simulink model "Transmitter_16bit"  (R2017a)
settings: Solver=FixedStepDiscrete  StartTime=0.0  StopTime=10  RelTol=1e-3
InitFcn:
  | numHeaderBits = 16;
  | %numPreambleBits = 250;
  | AGCBarkerSymbols = 160+28;
  | EQTrainingSymbols = 250;
  | CRCGeneratorLag = 34; % CRCLen + 2
  | 
  | %% AGC Preamble
  | B13bipolar = [0 0 0 0 0 2 2 0 0 2 0 2];
  | rep = [B13bipolar, B13bipolar(1:4)];
  | AGCBarker = repmat(rep,1,10);
  | % Second preamble part
  | B11bipolar = [0 0 0 2 2 2 0 2  2 0 2];
  | TimingBarker = [B11bipolar,B11bipolar,B11bipolar,B11bipolar(1:6)];
  | PreambleBarkersInts = [AGCBarker, TimingBarker];
  | % Convert integer into their bit representation
  | PreambleBarkersBits = zeros(1,length(PreambleBarkersInts)*2);
  | PreambleBarkersBits(1:2:end) = (PreambleBarkersInts==2);
  | 
  | % Constants
  | % First preamble part
  | B13bipolar = [0 0 0 0 0 2 2 0 0 2 0 2];
  | rep = [B13bipolar, B13bipolar(1:4)];
  | AGCBarker = repmat(rep,1,10);
  | % Second preamble part
  | B11bipolar = [0 0 0 2 2 2 0 2  2 0 2];
  | TimingBarker = [B11bipolar,B11bipolar,B11bipolar(1:6)];
  | PreambleBarkersInts = [AGCBarker, TimingBarker];
  | % Convert integer into their bit representation
  | PreambleBarkersBits = false(1,length(PreambleBarkersInts)*2);
  | PreambleBarkersBits(1:2:end) = logical(PreambleBarkersInts==2);
  | pLen = uint16(length(PreambleBarkersBits));
libraries: simulink x11, hdlsllib x5, dspsigops x4, commseqgen3 x3, commdigbbndpm3 x2, commcnvcod2 x1, commcrc2 x1, commfilt2 x1
settings Model: DataTypeOverride=Off  Creator=tcollins  LastModifiedBy=tcollins
settings DataIOCC: SaveOutput=off  SaveTime=off
settings OptimizationCC: BlockReduction=off  ConditionallyExecuteInputs=off  DefaultParameterBehavior=Inlined
settings DebuggingCC: AlgebraicLoopMsg=error  SingleTaskRateTransMsg=error
settings HardwareCC: ProdBitPerPointer=32  ProdBitPerSizeT=32  ProdBitPerPtrDiffT=32  ProdLargestAtomicFloat=None  ProdIntDivRoundTo=Undefined  ProdEndianess=Unspecified  ProdWordSize=32  ProdHWDeviceType=ASIC/FPGA->ASIC/FPGA  ProdEqTarget=off

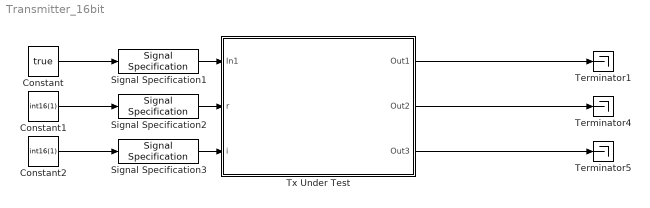
== system Transmitter_16bit ==
  Constant : Constant  Value=true  SampleTime=-1
  Constant1 : Constant  Value=int16(1)  SampleTime=-1
  Constant2 : Constant  Value=int16(1)  SampleTime=-1
  Signal Specification1 : SignalSpecification  OutDataTypeStr=boolean  SampleTime=1e-6
  Signal Specification2 : SignalSpecification  OutDataTypeStr=int16  SampleTime=1e-6
  Signal Specification3 : SignalSpecification  OutDataTypeStr=int16  SampleTime=1e-6
  Terminator1 : Terminator
  Terminator4 : Terminator
  Terminator5 : Terminator
  Tx Under Test : Subsystem  TreatAsAtomicUnit=on
  wires:
  Constant/1 -> Signal Specification1/1
  Tx Under Test/1(Out1) -> Terminator1/1
  Tx Under Test/2(Out2) -> Terminator4/1
  Tx Under Test/3(Out3) -> Terminator5/1
  Signal Specification1/1 -> Tx Under Test/1(In1)
  Constant1/1 -> Signal Specification2/1
  Signal Specification2/1 -> Tx Under Test/2("r ")
  Constant2/1 -> Signal Specification3/1
  Signal Specification3/1 -> Tx Under Test/3(i)

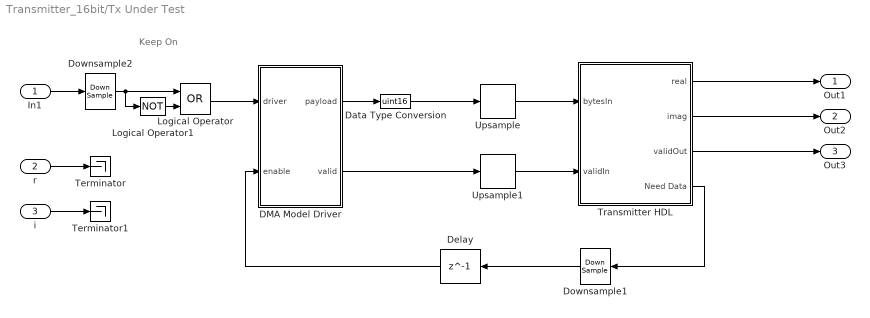
== system Transmitter_16bit/Tx Under Test ==
  note: Keep On
  In1 : Inport
  "r " : Inport  Port=2
  i : Inport  Port=3
  DMA Model Driver : MATLAB Function  TreatAsAtomicUnit=on
  Data Type Conversion : DataTypeConversion  OutDataTypeStr=uint16
  Delay : Delay  DelayLength=1
  Downsample1 : DownSample  N=4  RateOptions=Allow multirate processing
  Downsample2 : DownSample  N=4  RateOptions=Allow multirate processing
  Logical Operator : Logic  Operator=OR  AllPortsSameDT=off  OutDataTypeStr=boolean
  Logical Operator1 : Logic  Operator=NOT  AllPortsSameDT=off  OutDataTypeStr=boolean
  Terminator : Terminator
  Terminator1 : Terminator
  Transmitter HDL : Subsystem  TreatAsAtomicUnit=on
  Upsample : dspsigops/Upsample  N=4  phase=0  RateOptions=Allow multirate processing  ic=0  mode=Unused parameter value
  Upsample1 : dspsigops/Upsample  N=4  phase=0  RateOptions=Allow multirate processing  ic=0  mode=Unused parameter value
  Out1 : Outport
  Out2 : Outport  Port=2
  Out3 : Outport  Port=3
  wires:
  Transmitter HDL/4(Need Data) -> Downsample1/1
  Transmitter HDL/2(imag) -> Out2/1
  Transmitter HDL/1(real) -> Out1/1
  Transmitter HDL/3(validOut) -> Out3/1
  DMA Model Driver/1(payload) -> Data Type Conversion/1
  Delay/1 -> DMA Model Driver/2(enable)
  In1/1 -> Downsample2/1
  Data Type Conversion/1 -> Upsample/1
  DMA Model Driver/2(valid) -> Upsample1/1
  "r "/1 -> Terminator/1
  i/1 -> Terminator1/1
  Upsample/1 -> Transmitter HDL/1(bytesIn)
  Upsample1/1 -> Transmitter HDL/2(validIn)
  Downsample1/1 -> Delay/1
  Logical Operator/1 -> DMA Model Driver/1(driver)
  Logical Operator1/1 -> Logical Operator/2
  Downsample2/1 -> Logical Operator/1, Logical Operator1/1

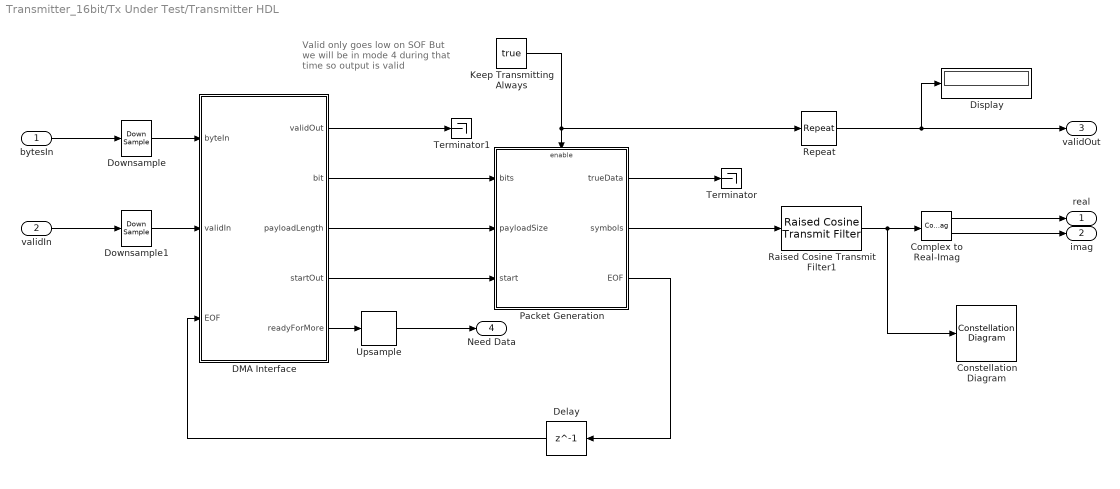
== system Transmitter_16bit/Tx Under Test/Transmitter HDL ==
  note: Valid only goes low on SOF
      | But we will be in mode 4 during
      | that time so output is valid
  bytesIn : Inport
  validIn : Inport  Port=2
  Complex to Real-Imag : ComplexToRealImag
  Constellation Diagram : ConstellationDiagram
  DMA Interface : Subsystem
  Delay : Delay  DelayLength=1
  Display : Display
  Downsample : DownSample  N=4  RateOptions=Allow multirate processing
  Downsample1 : DownSample  N=4  RateOptions=Allow multirate processing
  Keep Transmitting Always : Constant  Value=true  SampleTime=-1
  Packet Generation : Subsystem
  Raised Cosine Transmit Filter1 : commfilt2/Raised Cosine Transmit Filter  filtType=Square root  R=0.5  filtSpan=8  N=4  filterGain=1  RateOptions=Allow multirate processing  framing=Mute  checkCoeff=off  variableName=rcTxFilt1  checkGain=Normalized  sampMode=Mute  saveAsFlag=0  currentFiltSpan=8  D=(8)/2  launchFVT=on  roundingMode=Floor  overflowMode=off  coeffDataTypeStr=Inherit: Same word length as input  coeffMin=[]  coeffMax=[]  coeffLastDataTypeStr=Inherit: Same word length as input  outputMode=Binary point scaling  outputWordLength=16  outputFracLength=14  outputDataTypeStr=fixdt(1,16,14)  outputMin=[]  outputMax=[]  outputLastDataTypeStr=fixdt(1,16,14)
  Repeat : dspsigops/Repeat  N=4  InputProcessing=Columns as channels (frame based)  RateOptions=Allow multirate processing  ic=0  mode=Unused parameter value
      settings: SourceProductName=DSP System Toolbox
  Terminator : Terminator
  Terminator1 : Terminator
  Upsample : dspsigops/Upsample  N=4  phase=0  RateOptions=Allow multirate processing  ic=0  mode=Unused parameter value
  real : Outport
  imag : Outport  Port=2
  validOut : Outport  Port=3
  Need Data : Outport  Port=4
  wires:
  Raised Cosine Transmit Filter1/1 -> Constellation Diagram/1, Complex to Real-Imag/1
  Complex to Real-Imag/1 -> real/1
  Complex to Real-Imag/2 -> imag/1
  DMA Interface/2(bit) -> Packet Generation/1(bits)
  DMA Interface/3(payloadLength) -> Packet Generation/2(payloadSize)
  DMA Interface/4(startOut) -> Packet Generation/3(start)
  Packet Generation/2(symbols) -> Raised Cosine Transmit Filter1/1
  DMA Interface/5(readyForMore) -> Upsample/1
  Repeat/1 -> validOut/1, Display/1
  Packet Generation/1(trueData) -> Terminator/1
  Packet Generation/3(EOF) -> Delay/1
  Delay/1 -> DMA Interface/3(EOF)
  bytesIn/1 -> Downsample/1
  validIn/1 -> Downsample1/1
  Upsample/1 -> Need Data/1
  Downsample/1 -> DMA Interface/1(byteIn)
  Downsample1/1 -> DMA Interface/2(validIn)
  DMA Interface/1(validOut) -> Terminator1/1
  Keep Transmitting Always/1 -> Packet Generation/Enable, Repeat/1

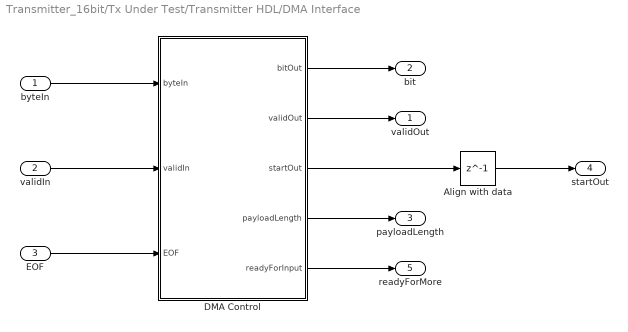
== system Transmitter_16bit/Tx Under Test/Transmitter HDL/DMA Interface ==
  byteIn : Inport
  validIn : Inport  Port=2
  EOF : Inport  Port=3
  Align with data : Delay  DelayLength=1
  DMA Control : MATLAB Function  TreatAsAtomicUnit=on
  validOut : Outport
  bit : Outport  Port=2
  payloadLength : Outport  Port=3  OutDataTypeStr=uint16
  startOut : Outport  Port=4
  readyForMore : Outport  Port=5
  wires:
  byteIn/1 -> DMA Control/1(byteIn)
  DMA Control/1(bitOut) -> bit/1
  DMA Control/5(readyForInput) -> readyForMore/1
  DMA Control/4(payloadLength) -> payloadLength/1
  DMA Control/2(validOut) -> validOut/1
  validIn/1 -> DMA Control/2(validIn)
  Align with data/1 -> startOut/1
  DMA Control/3(startOut) -> Align with data/1
  EOF/1 -> DMA Control/3(EOF)

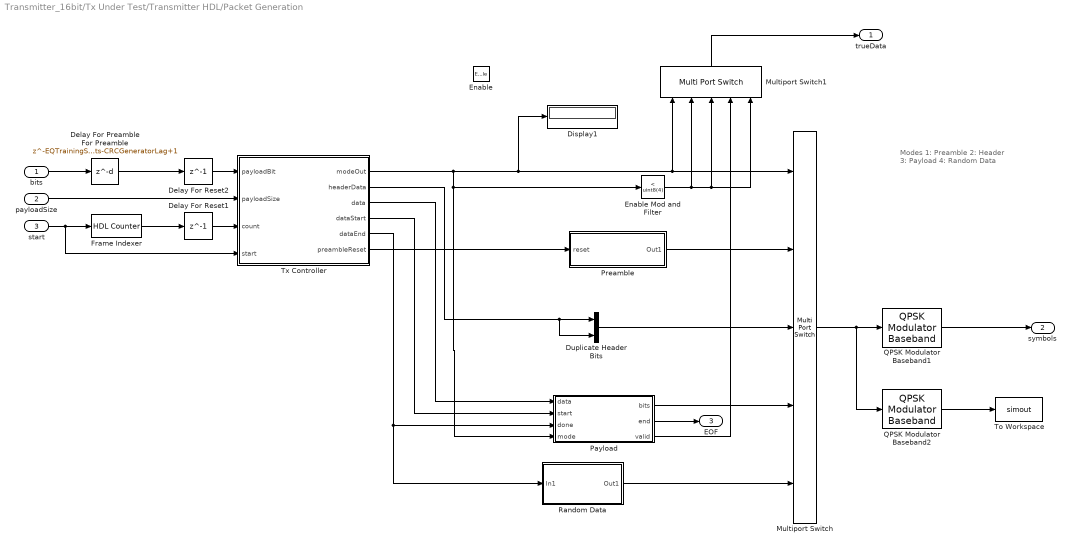
== system Transmitter_16bit/Tx Under Test/Transmitter HDL/Packet Generation ==
  note: Modes
      | 	1: Preamble
      | 	2: Header
      | 	3: Payload
      | 	4: Random Data
  bits : Inport  OutDataTypeStr=boolean
  payloadSize : Inport  Port=2
  start : Inport  Port=3
  Enable : EnablePort
  Delay For Preamble For Preamble : Delay  DelayLength=EQTrainingSymbols+AGCBarkerSymbols+numHeaderBits-CRCGeneratorLag+1  InitialCondition=false
  Delay For Reset1 : Delay  DelayLength=1
  Delay For Reset2 : Delay  DelayLength=1  InitialCondition=false
  Display1 : Display
  Duplicate Header Bits : Concatenate
  Enable Mod and Filter : simulink/Logic and Bit Operations/Compare To Constant  relop=<  const=uint8(4)  OutDataTypeStr=boolean
  Frame Indexer : hdlsllib/HDL Operations/HDL Counter  CountType=Count limited  CountInit=0  CountStep=1  CountMax=2^16+EQTrainingSymbols+AGCBarkerSymbols+numHeaderBits  CountFromType=Specify  CountFrom=0  CountResetPort=on  CountLoadPort=off  CountEnbPort=off  CountDirPort=off  CountDataType=Unsigned  CountWordLen=32  CountFracLen=0  CountSampTime=1
      settings: SourceProductName=HDL Coder  SourceProductBaseCode=HD
  Multiport Switch : MultiPortSwitch  Inputs=4
  Multiport Switch1 : MultiPortSwitch  Inputs=4
  Payload : Subsystem
  Preamble : Subsystem
  QPSK Modulator Baseband1 : commdigbbndpm3/QPSK Modulator Baseband  InType=Bit  Enc=Binary  Ph=pi/4  outDtype=Fixed-point  outWordLen=16  outUDDataType=sfix(16)  outFracLenMode=User-defined  outFracLen=15  outDataTypeStr=fixdt(1,16,15)  outLastDataTypeStr=fixdt(1,16,15)
  QPSK Modulator Baseband2 : commdigbbndpm3/QPSK Modulator Baseband  InType=Bit  Enc=Binary  Ph=pi/4  outDtype=double  outWordLen=16  outUDDataType=sfix(16)  outFracLenMode=User-defined  outFracLen=15  outDataTypeStr=double  outLastDataTypeStr=double
  Random Data : Subsystem
  To Workspace : ToWorkspace  VariableName=simout  SaveFormat=Timeseries  SampleTime=-1
  Tx Controller : MATLAB Function  TreatAsAtomicUnit=on
  trueData : Outport  InitialOutput=0
  symbols : Outport  Port=2  InitialOutput=complex(0)
  EOF : Outport  Port=3  OutDataTypeStr=boolean  InitialOutput=0
  wires:
  Tx Controller/2(headerData) -> Duplicate Header Bits/2, Duplicate Header Bits/1
  Random Data/1(Out1) -> Multiport Switch/5
  Enable Mod and Filter/1 -> Multiport Switch1/5, Multiport Switch1/3, Multiport Switch1/2
  Tx Controller/3(data) -> Payload/1(data)
  Tx Controller/4(dataStart) -> Payload/2(start)
  Delay For Preamble For Preamble/1 -> Delay For Reset2/1
  start/1 -> Tx Controller/4(start), Frame Indexer/1
  Preamble/1(Out1) -> Multiport Switch/2
  bits/1 -> Delay For Preamble For Preamble/1
  QPSK Modulator Baseband1/1 -> symbols/1
  Multiport Switch1/1 -> trueData/1
  Delay For Reset1/1 -> Tx Controller/3(count)
  Multiport Switch/1 -> QPSK Modulator Baseband2/1, QPSK Modulator Baseband1/1
  Tx Controller/5(dataEnd) -> Payload/3(done), Random Data/1(In1)
  Payload/1(bits) -> Multiport Switch/4
  Duplicate Header Bits/1 -> Multiport Switch/3
  Frame Indexer/1 -> Delay For Reset1/1
  Payload/3(valid) -> Multiport Switch1/4
  Payload/2(end) -> EOF/1
  payloadSize/1 -> Tx Controller/2(payloadSize)
  Tx Controller/1(modeOut) -> Display1/1, Multiport Switch/1, Multiport Switch1/1, Payload/4(mode), Enable Mod and Filter/1
  Tx Controller/6(preambleReset) -> Preamble/1(reset)
  Delay For Reset2/1 -> Tx Controller/1(payloadBit)
  QPSK Modulator Baseband2/1 -> To Workspace/1

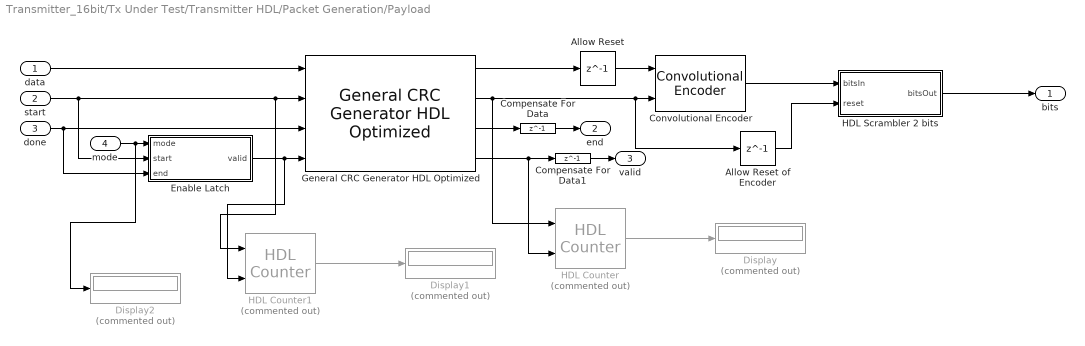
== system Transmitter_16bit/Tx Under Test/Transmitter HDL/Packet Generation/Payload ==
  data : Inport
  start : Inport  Port=2
  done : Inport  Port=3
  mode : Inport  Port=4
  Allow Reset : Delay  DelayLength=1
  Allow Reset of Encoder : Delay  DelayLength=1
  Compensate For Data : Delay  DelayLength=1
  Compensate For Data1 : Delay  DelayLength=1
  Convolutional Encoder : commcnvcod2/Convolutional Encoder  trellis=poly2trellis(7, [171 133])  opMode=Reset on nonzero input via port  DelayedResetAction=on  hasIniStPort=off  hasFinStPort=off  usePuncVector=off  punctureVector=[1; 1; 0; 1; 0; 1]  reset=Unused parameter value
      settings: SourceProductName=Communications System Toolbox  SourceProductBaseCode=CM
  Display : Display  Commented=on
  Display1 : Display  Commented=on
  Display2 : Display  Commented=on
  Enable Latch : Subsystem
  General CRC Generator HDL Optimized : commcrc2/General CRC Generator HDL Optimized  Polynomial=[1 0 0 0 0 0 1 0 0 1 1 0 0 0 0 0 1 0 0 0 1 1 1 0 1 1 0 1 1 0 1 1 1]  InitialState=0  DirectMethod=off  ReflectInput=off  ReflectCRCChecksum=off  FinalXORValue=0  SimulateUsing=Code generation
      settings: SourceProductName=Communications System Toolbox  SourceProductBaseCode=CM
  HDL Counter : hdlsllib/HDL Operations/HDL Counter  Commented=on  CountType=Count limited  CountInit=0  CountStep=1  CountMax=1e4  CountFromType=Initial value  CountFrom=0  CountResetPort=on  CountLoadPort=off  CountEnbPort=on  CountDirPort=off  CountDataType=Unsigned  CountWordLen=16  CountFracLen=0  CountSampTime=1
      settings: SourceProductName=HDL Coder  SourceProductBaseCode=HD
  HDL Counter1 : hdlsllib/HDL Operations/HDL Counter  Commented=on  CountType=Count limited  CountInit=0  CountStep=1  CountMax=1e4  CountFromType=Initial value  CountFrom=0  CountResetPort=on  CountLoadPort=off  CountEnbPort=on  CountDirPort=off  CountDataType=Unsigned  CountWordLen=16  CountFracLen=0  CountSampTime=1
      settings: SourceProductName=HDL Coder  SourceProductBaseCode=HD
  HDL Scrambler 2 bits : Subsystem  mask{poly=[1 1 0 1 0 1 0 1], init_state=[0 1 0 0 0 1 0]}
      mask prompts: poly "Polynomial"; init_state "Initial State"
  bits : Outport
  end : Outport  Port=2
  valid : Outport  Port=3
  wires:
  General CRC Generator HDL Optimized/1 -> Allow Reset/1
  data/1 -> General CRC Generator HDL Optimized/1
  start/1 -> Enable Latch/2(start), HDL Counter1/1, General CRC Generator HDL Optimized/2
  General CRC Generator HDL Optimized/4 -> HDL Counter/2, Compensate For Data1/1
  done/1 -> Enable Latch/3(end), General CRC Generator HDL Optimized/3
  mode/1 -> Display2/1, Enable Latch/1(mode)
  Convolutional Encoder/1 -> HDL Scrambler 2 bits/1(bitsIn)
  General CRC Generator HDL Optimized/2 -> HDL Counter/1, Allow Reset of Encoder/1, Convolutional Encoder/2
  HDL Scrambler 2 bits/1(bitsOut) -> bits/1
  Enable Latch/1(valid) -> HDL Counter1/2, General CRC Generator HDL Optimized/4
  Allow Reset/1 -> Convolutional Encoder/1
  General CRC Generator HDL Optimized/3 -> Compensate For Data/1
  Allow Reset of Encoder/1 -> HDL Scrambler 2 bits/2(reset)
  HDL Counter/1 -> Display/1
  HDL Counter1/1 -> Display1/1
  Compensate For Data/1 -> end/1
  Compensate For Data1/1 -> valid/1

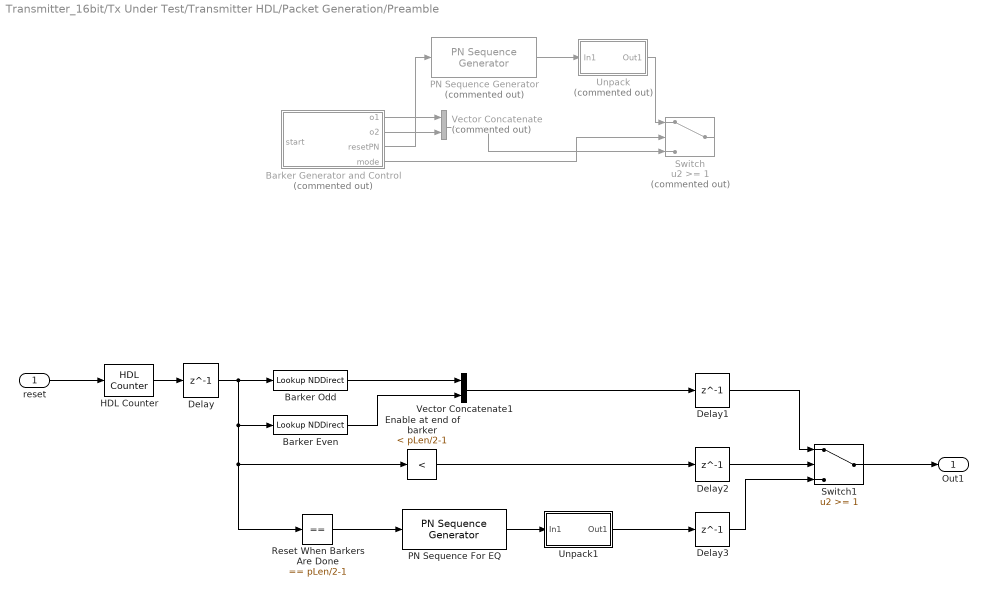
== system Transmitter_16bit/Tx Under Test/Transmitter HDL/Packet Generation/Preamble ==
  reset : Inport
  Barker Even : LookupNDDirect  NumberOfTableDimensions=1  Table=[PreambleBarkersBits(4:2:end),false(1,400)]  DiagnosticForOutOfRangeInput=Error  TableDataTypeStr=boolean
  Barker Generator and Control : MATLAB Function  Commented=on  TreatAsAtomicUnit=on
  Barker Odd : LookupNDDirect  NumberOfTableDimensions=1  Table=[PreambleBarkersBits(3:2:end-1),false(1,400)]  DiagnosticForOutOfRangeInput=Error  TableDataTypeStr=boolean
  Delay{,1..3} (4 alike) : Delay  DelayLength=1
  Enable at end of barker : simulink/Logic and Bit Operations/Compare To Constant  relop=<  const=pLen/2-1  OutDataTypeStr=boolean
  HDL Counter : hdlsllib/HDL Operations/HDL Counter  CountType=Count limited  CountInit=0  CountStep=1  CountMax=pLen/2-2+400  CountFromType=Initial value  CountFrom=0  CountResetPort=on  CountLoadPort=off  CountEnbPort=off  CountDirPort=off  CountDataType=Unsigned  CountWordLen=16  CountFracLen=0  CountSampTime=1
      settings: SourceProductName=HDL Coder  SourceProductBaseCode=HD
  PN Sequence For EQ : commseqgen3/PN Sequence Generator  poly='z^5 + z^3 + z^1 + 1'  ini_sta=[1 1 1 0 0]  outBitMaskSource=Dialog parameter  shift=0  outVarSiz=off  maxOutSizeMode=Dialog parameter  maxOutSize=[10 1]  Ts=-1  sampPerFrame=1  reset=on  bitPackedOutputs=on  outDataType=double  numPackedBits=2  bitPackDataSigned=off  bitPackedOutDType=Smallest integer
      settings: SourceProductName=Communications System Toolbox
  PN Sequence Generator : commseqgen3/PN Sequence Generator  Commented=on  poly='z^3 + z^2 + 1'  ini_sta=[0 0 1]  outBitMaskSource=Dialog parameter  shift=0  outVarSiz=off  maxOutSizeMode=Dialog parameter  maxOutSize=[10 1]  Ts=-1  sampPerFrame=1  reset=on  bitPackedOutputs=on  outDataType=double  numPackedBits=2  bitPackDataSigned=off  bitPackedOutDType=Smallest integer
      settings: SourceProductName=Communications System Toolbox
  Reset When Barkers Are Done : simulink/Logic and Bit Operations/Compare To Constant  relop===  const=pLen/2-1  OutDataTypeStr=boolean
  Switch : Switch  Commented=on  Threshold=1
  Switch1 : Switch  Threshold=1
  Unpack : Subsystem  Commented=on
  Unpack1 : Subsystem
  Vector Concatenate : Concatenate  Commented=on
  Vector Concatenate1 : Concatenate
  Out1 : Outport
  wires:
  reset/1 -> HDL Counter/1
  Barker Odd/1 -> Vector Concatenate1/1
  Barker Even/1 -> Vector Concatenate1/2
  PN Sequence For EQ/1 -> Unpack1/1(In1)
  Switch1/1 -> Out1/1
  Reset When Barkers Are Done/1 -> PN Sequence For EQ/1
  Barker Generator and Control/3(resetPN) -> PN Sequence Generator/1
  Barker Generator and Control/1(o1) -> Vector Concatenate/1
  Barker Generator and Control/4(mode) -> Switch/2
  PN Sequence Generator/1 -> Unpack/1(In1)
  Barker Generator and Control/2(o2) -> Vector Concatenate/2
  Unpack/1(Out1) -> Switch/1
  Vector Concatenate/1 -> Switch/3
  ? -> Barker Generator and Control/1(start)
  HDL Counter/1 -> Delay/1
  Delay/1 -> Enable at end of barker/1, Reset When Barkers Are Done/1, Barker Even/1, Barker Odd/1
  Vector Concatenate1/1 -> Delay1/1
  Enable at end of barker/1 -> Delay2/1
  Unpack1/1(Out1) -> Delay3/1
  Delay1/1 -> Switch1/1
  Delay2/1 -> Switch1/2
  Delay3/1 -> Switch1/3

== system Transmitter_16bit/Tx Under Test/Transmitter HDL/Packet Generation/Random Data ==
  In1 : Inport
  Random Data Gen : commseqgen3/PN Sequence Generator  poly='z^3 + z^2 + 1'  ini_sta=[0 0 1]  outBitMaskSource=Dialog parameter  shift=0  outVarSiz=off  maxOutSizeMode=Dialog parameter  maxOutSize=[10 1]  Ts=-1  sampPerFrame=1  reset=on  bitPackedOutputs=on  outDataType=double  numPackedBits=2  bitPackDataSigned=off  bitPackedOutDType=Smallest integer
      settings: SourceProductName=Communications System Toolbox
  Unpack : Subsystem
  Out1 : Outport
  wires:
  In1/1 -> Random Data Gen/1
  Unpack/1(Out1) -> Out1/1
  Random Data Gen/1 -> Unpack/1(In1)

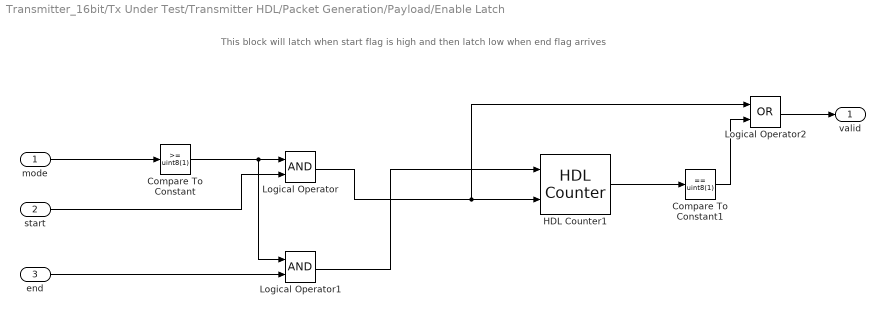
== system Transmitter_16bit/Tx Under Test/Transmitter HDL/Packet Generation/Payload/Enable Latch ==
  note: This block will latch when start flag is high and then latch low when end flag arrives
  mode : Inport
  start : Inport  Port=2
  end : Inport  Port=3
  Compare To Constant : simulink/Logic and Bit Operations/Compare To Constant  relop=>=  const=uint8(1)  OutDataTypeStr=boolean
  Compare To Constant1 : simulink/Logic and Bit Operations/Compare To Constant  relop===  const=uint8(1)  OutDataTypeStr=boolean
  HDL Counter1 : hdlsllib/HDL Operations/HDL Counter  CountType=Count limited  CountInit=0  CountStep=1  CountMax=1  CountFromType=Initial value  CountFrom=0  CountResetPort=on  CountLoadPort=off  CountEnbPort=on  CountDirPort=off  CountDataType=Unsigned  CountWordLen=8  CountFracLen=0  CountSampTime=1
      settings: SourceProductName=HDL Coder  SourceProductBaseCode=HD
  Logical Operator : Logic  AllPortsSameDT=off  OutDataTypeStr=boolean
  Logical Operator1 : Logic  AllPortsSameDT=off  OutDataTypeStr=boolean
  Logical Operator2 : Logic  Operator=OR  AllPortsSameDT=off  OutDataTypeStr=boolean
  valid : Outport
  wires:
  mode/1 -> Compare To Constant/1
  Compare To Constant/1 -> Logical Operator1/1, Logical Operator/1
  start/1 -> Logical Operator/2
  end/1 -> Logical Operator1/2
  HDL Counter1/1 -> Compare To Constant1/1
  Logical Operator1/1 -> HDL Counter1/1
  Logical Operator/1 -> Logical Operator2/1, HDL Counter1/2
  Compare To Constant1/1 -> Logical Operator2/2
  Logical Operator2/1 -> valid/1

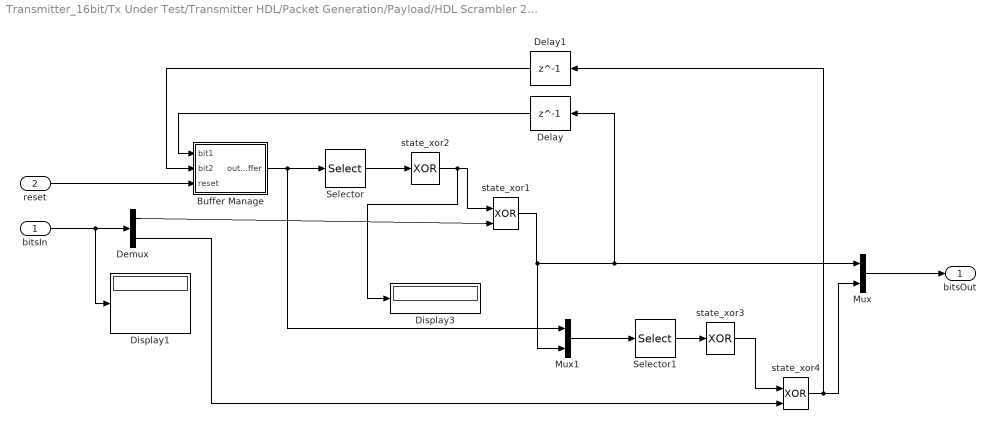
== system Transmitter_16bit/Tx Under Test/Transmitter HDL/Packet Generation/Payload/HDL Scrambler 2 bits ==
  bitsIn : Inport
  reset : Inport  Port=2
  Buffer Manage : MATLAB Function  TreatAsAtomicUnit=on
  Delay : Delay  DelayLength=1  InitialCondition=false
  Delay1 : Delay  DelayLength=1  InitialCondition=false
  Demux : Demux  Outputs=2
  Display1 : Display
  Display3 : Display
  Mux : Mux  Inputs=2
  Mux1 : Mux  Inputs=2
  Selector : Selector  IndexOptions=Index vector (dialog)  Indices=find(poly(2:end))  OutputSizes=1
  Selector1 : Selector  IndexOptions=Index vector (dialog)  Indices=1+find(poly(2:end))  OutputSizes=1
  state_xor1 : Logic  Operator=XOR  IconShape=distinctive  AllPortsSameDT=off  OutDataTypeStr=boolean
  state_xor2 : Logic  Operator=XOR  Inputs=1  IconShape=distinctive  AllPortsSameDT=off  OutDataTypeStr=boolean
  state_xor3 : Logic  Operator=XOR  Inputs=1  IconShape=distinctive  AllPortsSameDT=off  OutDataTypeStr=boolean
  state_xor4 : Logic  Operator=XOR  IconShape=distinctive  AllPortsSameDT=off  OutDataTypeStr=boolean
  bitsOut : Outport
  wires:
  bitsIn/1 -> Display1/1, Demux/1
  Selector/1 -> state_xor2/1
  state_xor2/1 -> Display3/1, state_xor1/1
  Demux/1 -> state_xor1/2
  state_xor1/1 -> Mux1/2, Mux/1, Delay/1
  Mux/1 -> bitsOut/1
  Mux1/1 -> Selector1/1
  Buffer Manage/1(outBuffer) -> Mux1/1, Selector/1
  Selector1/1 -> state_xor3/1
  state_xor3/1 -> state_xor4/1
  Demux/2 -> state_xor4/2
  state_xor4/1 -> Delay1/1, Mux/2
  Delay/1 -> Buffer Manage/1(bit1)
  reset/1 -> Buffer Manage/3(reset)
  Delay1/1 -> Buffer Manage/2(bit2)

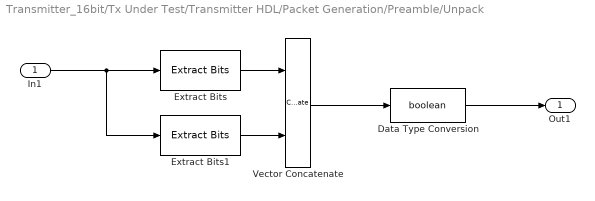
== system Transmitter_16bit/Tx Under Test/Transmitter HDL/Packet Generation/Preamble/Unpack ==
  In1 : Inport
  Data Type Conversion : DataTypeConversion  OutDataTypeStr=boolean
  Extract Bits : simulink/Logic and Bit Operations/Extract Bits  bitsToExtract=Range of bits  numBits=8  bitIdxRange=[1]  outScalingMode=Treat bit field as an integer
      settings: SourceProductName=Simulink
  Extract Bits1 : simulink/Logic and Bit Operations/Extract Bits  bitsToExtract=Range of bits  numBits=8  bitIdxRange=[0]  outScalingMode=Treat bit field as an integer
      settings: SourceProductName=Simulink
  Vector Concatenate : Concatenate
  Out1 : Outport
  wires:
  In1/1 -> Extract Bits1/1, Extract Bits/1
  Extract Bits/1 -> Vector Concatenate/1
  Extract Bits1/1 -> Vector Concatenate/2
  Vector Concatenate/1 -> Data Type Conversion/1
  Data Type Conversion/1 -> Out1/1

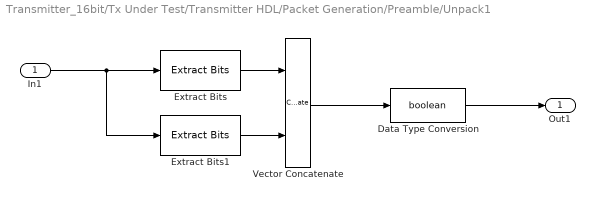
== system Transmitter_16bit/Tx Under Test/Transmitter HDL/Packet Generation/Preamble/Unpack1 ==
  In1 : Inport
  Data Type Conversion : DataTypeConversion  OutDataTypeStr=boolean
  Extract Bits : simulink/Logic and Bit Operations/Extract Bits  bitsToExtract=Range of bits  numBits=8  bitIdxRange=[1]  outScalingMode=Treat bit field as an integer
      settings: SourceProductName=Simulink
  Extract Bits1 : simulink/Logic and Bit Operations/Extract Bits  bitsToExtract=Range of bits  numBits=8  bitIdxRange=[0]  outScalingMode=Treat bit field as an integer
      settings: SourceProductName=Simulink
  Vector Concatenate : Concatenate
  Out1 : Outport
  wires:
  In1/1 -> Extract Bits1/1, Extract Bits/1
  Extract Bits/1 -> Vector Concatenate/1
  Extract Bits1/1 -> Vector Concatenate/2
  Vector Concatenate/1 -> Data Type Conversion/1
  Data Type Conversion/1 -> Out1/1

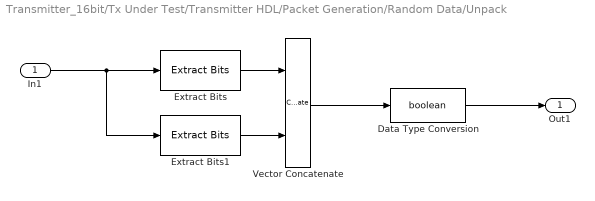
== system Transmitter_16bit/Tx Under Test/Transmitter HDL/Packet Generation/Random Data/Unpack ==
  In1 : Inport
  Data Type Conversion : DataTypeConversion  OutDataTypeStr=boolean
  Extract Bits : simulink/Logic and Bit Operations/Extract Bits  bitsToExtract=Range of bits  numBits=8  bitIdxRange=[0]  outScalingMode=Treat bit field as an integer
      settings: SourceProductName=Simulink
  Extract Bits1 : simulink/Logic and Bit Operations/Extract Bits  bitsToExtract=Range of bits  numBits=8  bitIdxRange=[1]  outScalingMode=Treat bit field as an integer
      settings: SourceProductName=Simulink
  Vector Concatenate : Concatenate
  Out1 : Outport
  wires:
  In1/1 -> Extract Bits1/1, Extract Bits/1
  Extract Bits/1 -> Vector Concatenate/1
  Extract Bits1/1 -> Vector Concatenate/2
  Vector Concatenate/1 -> Data Type Conversion/1
  Data Type Conversion/1 -> Out1/1

== matlab function Transmitter_16bit/Tx Under Test/Transmitter HDL/Packet Generation/Preamble/Barker Generator and Control ==
  data: start input; o1 output; o2 output; resetPN output; mode output
function [o1,o2,resetPN,mode] = fcn(start)

persistent indx

% Constants
% First preamble part
B13bipolar = [0 0 0 0 0 2 2 0 0 2 0 2];
rep = [B13bipolar, B13bipolar(1:4)];
AGCBarker = repmat(rep,1,10);
% Second preamble part
B11bipolar = [0 0 0 2 2 2 0 2  2 0 2];
TimingBarker = [B11bipolar,B11bipolar,B11bipolar(1:6)];
PreambleBarkersInts = [AGCBarker, TimingBarker];
% Convert integer into their bit representation
PreambleBarkersBits = false(1,length(PreambleBarkersInts)*2);
PreambleBarkersBits(1:2:end) = logical(PreambleBarkersInts==2);
pLen = uint16(length(PreambleBarkersBits));

% Async
if isempty(indx)
       indx = uint16(3);
end

% Reset and Async
if start
    resetPN = false; % Not important
    indx = uint16(3);
    o1 = PreambleBarkersBits(1);
    o2 = PreambleBarkersBits(2);
    mode = uint8(0); % Barker
else
    % Preamble is done, now PN can go
    if indx==(pLen+uint16(1))
        indx = indx + uint16(2); % Push last if to else
        resetPN = true;
    else
        resetPN = false;
    end
    % mode -> 0==Barkers | 1==PN
    if indx<(pLen)
        o1 = PreambleBarkersBits(indx);
        o2 = PreambleBarkersBits(indx+1);
        indx = indx + uint16(2);
        mode = uint8(0); % Barker
    else
        o1 = false;
        o2 = false;
        mode = uint8(1);
    end

%     if indx<pLen
%         o1 = PreambleBarkersBits(indx);
%         o2 = PreambleBarkersBits(indx+1);
%         indx = indx + uint16(2);
%         mode = uint8(0); % Barker
    
    
    
    
end

== matlab function Transmitter_16bit/Tx Under Test/Transmitter HDL/Packet Generation/Tx Controller ==
  data: modeOut output; headerData output; data output; payloadBit input; payloadSize input; count input; start input; dataStart output; dataEnd output; preambleReset output
function [modeOut, headerData, data, dataStart, dataEnd, preambleReset] = fcn(payloadBit,payloadSize,count, start)

% When we get a start flag buffers are reset and the next cycle with start
% in mode 0

% Reset: New payload size is passed at an int16
% 


persistent  headerBits numPayloadBits mode

numHeaderBits = uint32(16);
AGCBarkerSymbols = 160+28;
EQTrainingSymbols = 250; % 2 bits per symbol => 250 symbols
preambleBits = uint32(EQTrainingSymbols+AGCBarkerSymbols-0);
CRCLength = 32;
CRCGeneratorLag = CRCLength+2+0; % additional 1 is from reset of encoder
CodeRate = 2;
lagBits = 40+68;

% Async/Init
if isempty(numPayloadBits)
    % Sizes of frame sections
    numPayloadBits = uint32(0); 
    %headerBits = zeros(1,numHeaderBits)>0;
    headerBits = uint16(0);
    mode = uint8(4);
end

% Synchronous
switch mode
    case uint8(0) % Reset
        % Move to next mode on next input/clock
        mode = uint8(1);
        % Convert payloadSize to bits
        numPayloadBits = uint32(bitshift(payloadSize,3)+CRCLength);
        %headerBits = logical(bitget(CodeRate*(payloadSize+CRCLength),1:numHeaderBits));
        headerBits = uint16(bitshift((bitshift(payloadSize,3)+CRCLength+lagBits),1));        
        % Set outputs
        modeOut = uint8(4);
        headerData = false;
        data = false; % Not used downstream
        dataStart = false;
        dataEnd = false;
        preambleReset = true;
    case uint8(1) % Preamble
        % Set Next Mode
        if count>=(preambleBits)
            preambleReset = false;
            mode = uint8(2);
        elseif count==uint32(1)
            preambleReset = false;
            mode = uint8(1);
        else
            preambleReset = false;
            mode = uint8(1);
        end
        % Set outputs
        modeOut = uint8(1);
        headerData = false;
        % Start outputing data early to compensate for CRC lag
        if count>=(preambleBits+numHeaderBits-CRCGeneratorLag)
           data = payloadBit;
           % Set flag on first payload bit
           dataStart = count == (preambleBits+numHeaderBits-CRCGeneratorLag);
        else
           data = false;         
           dataStart = false;
        end
        dataEnd = false;
    case uint8(2) % Header bits
        % Set Next Mode
        if count>=(preambleBits+numHeaderBits)
            mode = uint8(3);
        else
            mode = uint8(2);
        end
        % Set outputs
        modeOut = uint8(2);
        %headerData = headerBits(count-preambleBits);
        headerData = bitget(headerBits,count-preambleBits)>0;
        data = payloadBit;
        dataStart = false;
        dataEnd = false;
        preambleReset = false;
    case uint8(3) % Payload bits and CRC
        % Set Next Mode
        if count>=(preambleBits+numHeaderBits+numPayloadBits)%+CRCGeneratorLag)
            % Will coencide with last CRC Bit
            mode = uint8(4);
        else
            mode = uint8(3);
        end
        % Set outputs
        modeOut = uint8(3);        
        headerData = false;
        data = payloadBit;
        % Set flag on last payload bit
        dataStart = false;
        dataEnd =   ( count==(preambleBits+numHeaderBits+numPayloadBits-CRCLength-CRCGeneratorLag-1) );
        preambleReset = false;
    otherwise %case uint8(4) % Waiting for data
        % Chilling for new start
        if start
           mode = uint8(0); 
        else
           mode = uint8(4);
        end
        % Set outputs
        modeOut = uint8(4);
        headerData = false;
        data = false; % Not used downstream
        dataStart = false;
        dataEnd = false;
        preambleReset = false;
end

== matlab function Transmitter_16bit/Tx Under Test/Transmitter HDL/DMA Interface/DMA Control ==
  data: byteIn input; bitOut output; validIn input; validOut output; startOut output; payloadLength output; readyForInput output; EOF input
function [bitOut,validOut,startOut,payloadLength,readyForInput] = DMA_Control(byteIn,validIn,EOF)

% This block converts the byte input pipeline into bits and extract the
% length the packet into its own signal

persistent wordBuffer bitCounter payloadLenBuff mode inputByteCounter

bitsInInput = uint8(16);
bytesInInput = uint16(2);

if isempty(wordBuffer)
    wordBuffer = uint16(0); % Must match number of bits defined by bitsInInput
    bitCounter = uint8(0);
    payloadLenBuff = uint16(0);
    mode = uint8(0);
    inputByteCounter = uint16(0);
end

%% Payload length setup
% Capture first payload length byte(s)
if validIn && mode == uint8(0)
    mode = uint8(2);
    payloadLenBuff = uint16(byteIn);
    % Set outputs
    bitOut = false;
    validOut = false;
    startOut = true;
    payloadLength = uint16(0);
    readyForInput = true;
    % Reset counters
    inputByteCounter = bytesInInput;% Reset
    bitCounter = uint8(1);% Reset
    
%% Payload output
elseif (bitCounter > uint8(0))  && (mode==uint8(2))
    % Set outputs
    if bitCounter==uint8(1)
        bitOut = bitget(byteIn,1)>0;
        wordBuffer = byteIn; % Save byte
    else
        bitOut = bitget(wordBuffer,bitCounter)>0;
    end
    startOut = false;
    payloadLength = uint16(payloadLenBuff);
    validOut = true;
    % Set flag to DMA and next mode
    if bitCounter >= uint8(bitsInInput)
        bitCounter = uint8(1); % Reset
        % If we've processed all the bytes we need to wait for downstream
        % to be done
        if inputByteCounter<payloadLenBuff
            readyForInput = true; % Tell them we need next byte
            % Bytes processed
            inputByteCounter = inputByteCounter + bytesInInput;    
        else
            readyForInput = false; % Hold DMA off for now, next call will go to EOF
            mode = uint8(3);
        end
    else
        bitCounter = bitCounter+uint8(1);
        readyForInput = false;
    end
% Waiting for EOF from packet generation
elseif (mode==uint8(3))
    bitOut = false;
    validOut = true; % Keep downstream processing going
    startOut = false;
    payloadLength = uint16(payloadLenBuff);
    if EOF % Done with frame now ask for more data
        readyForInput = true;
        mode = uint8(0);% Reset
    else
        readyForInput = false;
    end
    
else % not-valid and need another byte
    bitOut = false;
    if mode == uint8(0)
        validOut = true; % Let LFSR Run
    else
        validOut = false;
    end
    startOut = false;
    payloadLength = uint16(0);
    readyForInput = true;
end

== matlab function Transmitter_16bit/Tx Under Test/Transmitter HDL/Packet Generation/Payload/HDL Scrambler 2 bits/Buffer Manage ==
  data: bit1 input; bit2 input; outBuffer output; reset input
function outBuffer = fcn(bit1, bit2, reset)
%#codegen

init_buffer = logical([0 1 0 0 0 1 0]);

persistent buffer

if isempty(buffer)
    buffer = init_buffer;
end

if reset
    outBuffer = init_buffer;
    buffer = init_buffer;
    %outBuffer = [init_buffer(3:end),bit1,bit2];
    %buffer = [buffer(3:end),bit1,bit2];    
else
    outBuffer = [bit2,bit1,buffer(1:end-2)];
    buffer = [bit2,bit1,buffer(1:end-2)];
end

== matlab function Transmitter_16bit/Tx Under Test/DMA Model Driver ==
  data: driver input; payload output; valid output boolean; enable input
function [payload,valid] = fcn(driver, enable)
%#codegen

persistent indx mode

pSize = uint16(200); % Size in bytes (Must be multiple of 32 bits) cannot exceed uint16 max
mask = uint16(sum(2.^(0:15)));

if isempty(indx)
    indx = pSize;
    mode = int8(0);
end

% % Randomly dont transmit new data
% if enable && mode == 0
%    enable = randn>1; 
% end

if enable && driver
    valid = true;
    switch mode
        case int8(0) % Fresh packet start
%             disp('New Packet Start');
            payload = uint16(pSize);%Upper bits
            mode = int8(1);
            indx = uint16(0);
        otherwise%case 2
            indx = indx + uint16(2);
            if indx == uint16(2)
                payload = uint16(0);
            elseif indx == pSize
                payload = uint16(2^16-1); % All ones
            else
                payload = uint16(21845*2);%sum(2.^[0:2:14])); % Alternating ones and zeros
            end
            
            if indx == pSize % reached end of frame
                mode = int8(0);
            end
    end
else
    valid = false;
    payload = uint16(0);
end
